simulink model "roomheating"  (Simulink 8.3)
settings: Solver=ode45  StartTime=0.0  StopTime=6  FixedStep=0.000017  RelTol=1e-3
settings Model: Creator=yangg  LastModifiedBy=yangg
settings DataIOCC: MaxDataPoints=1000000  SaveFormat=StructureWithTime
settings OptimizationCC: ExpressionDepthLimit=2147483647
settings DebuggingCC: FcnCallInpInsideContextMsg=EnableAllAsWarning
settings GRTTargetCC: CombineOutputUpdateFcns=on  GRTInterface=off

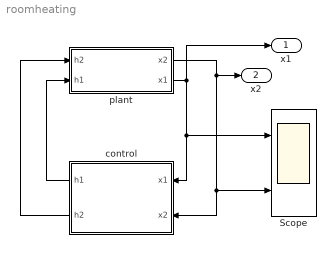
== system roomheating ==
  Scope : Scope  NumInputPorts=2
      settings: TimeRange=0.09  YMin=19.998~99.997  YMax=20.003~100.004  MaxDataPoints=999999999
  control : Stateflow chart  TreatAsAtomicUnit=on
  plant : Subsystem
  x1 : Outport  SampleTime=0
  x2 : Outport  Port=2  SampleTime=0
  wires:
  control/1(h1) -> plant/2(h1)
  control/2(h2) -> plant/1(h2)
  plant/1(x2) -> x2/1, Scope/2, control/2(x2)
  plant/2(x1) -> Scope/1, control/1(x1), x1/1

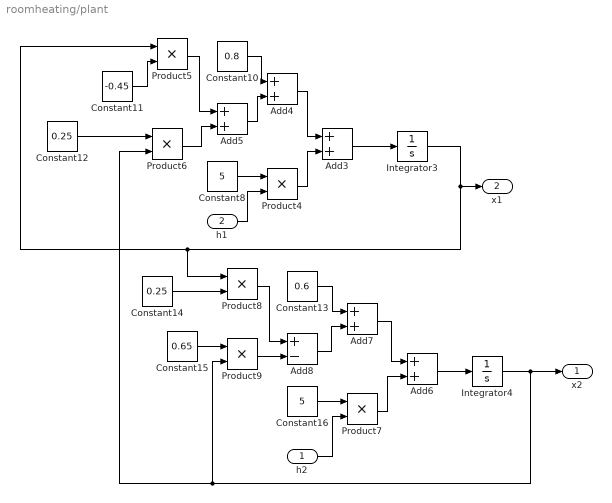
== system roomheating/plant ==
  h2 : Inport  SampleTime=0.001
  h1 : Inport  Port=2  SampleTime=0.001
  Add{3..7} (5 alike) : Sum  SampleTime=0.001
  Add8 : Sum  Inputs=+-  SampleTime=0.001
  Constant10 : Constant  Value=0.8
  Constant11 : Constant  Value=-0.45
  Constant12 : Constant  Value=0.25
  Constant13 : Constant  Value=0.6
  Constant14 : Constant  Value=0.25
  Constant15 : Constant  Value=0.65
  Constant16 : Constant  Value=5
  Constant8 : Constant  Value=5
  Integrator3 : Integrator  InitialCondition=10
  Integrator4 : Integrator  InitialCondition=10
  Product{4..9} (6 alike) : Product  SampleTime=0.001  RndMeth=Zero
  x2 : Outport  SampleTime=0.0001
  x1 : Outport  Port=2  SampleTime=0.0001
  wires:
  Constant8/1 -> Product4/1
  h1/1 -> Product4/2
  Product4/1 -> Add3/2
  Add3/1 -> Integrator3/1
  Integrator3/1 -> Product8/1, Product5/1, x1/1
  Add4/1 -> Add3/1
  Constant10/1 -> Add4/1
  Add5/1 -> Add4/2
  Product5/1 -> Add5/1
  Product6/1 -> Add5/2
  Constant11/1 -> Product5/2
  Constant12/1 -> Product6/1
  Constant16/1 -> Product7/1
  h2/1 -> Product7/2
  Product7/1 -> Add6/2
  Add6/1 -> Integrator4/1
  Integrator4/1 -> Product6/2, Product9/2, x2/1
  Add7/1 -> Add6/1
  Constant13/1 -> Add7/1
  Add8/1 -> Add7/2
  Product8/1 -> Add8/1
  Product9/1 -> Add8/2
  Constant14/1 -> Product8/2
  Constant15/1 -> Product9/1

== stateflow chart control ==
  settings: updateMethod=DISCRETE  sampleTime=0.1
  state room1_on
    entry:
    h1=1;
    h2=0;
  state changeto2
    entry:
    owner=2;
    h1=0;
    h2=1;
  state room1_off
    entry:
    h1=0;
  state decide
  state changeto1
    entry:
    owner=1;
    h1=1;
    h2=0;
  state room2_on
    entry:
    h1=0;
    h2=1;
  state room2_off
    entry:
    h2=0;
  (default) -> decide : /owner=1
  decide -> room1_on [order 5] : [x1<=10&&owner==1]
  decide -> room2_on [order 3] : [x2<=10&&owner==2]
  room1_on -> decide
  room2_on -> decide
  decide -> room1_off [order 6] : [x1>=12]
  decide -> room2_off [order 4] : [x2>=12]
  room1_off -> decide
  room2_off -> decide
  decide -> changeto2 [order 1] : [owner==1&&x2<=8&&x1-x2>=0.5]
  changeto2 -> decide
  changeto1 -> decide
  decide -> changeto1 [order 2] : [owner==2&&x1<=8&&x2-x1>=0.5]
  data: x1 input double; x2 input double; h1 output double =1; h2 output double =0; owner local double
